simulink model "SO_SMC"  (R2023b)
settings: Solver=ode1  StartTime=0.0  StopTime=60  FixedStep=0.01  RelTol=1e-3
libraries: simulink x1
settings Model: Creator=vanch  LastModifiedBy=vanch

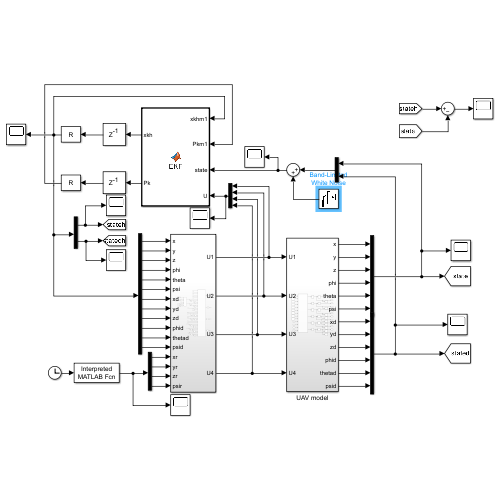
[thumbnail: Simulink's stored preview of the top-level diagram]
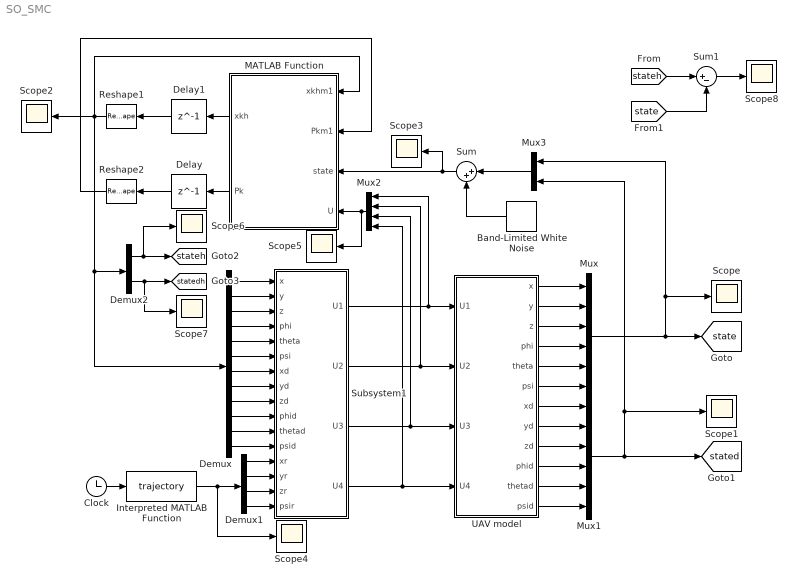
== system SO_SMC ==
  Band-Limited White Noise : simulink/Sources/Band-Limited White Noise  Cov=1e-8  Ts=0.01  seed=[1530]
  Clock : Clock
  Delay : Delay  DelayLength=1  InitialCondition=(1e-3)*eye(12,12)
  Delay1 : Delay  DelayLength=1  InitialCondition=0.001
  Demux : Demux  Outputs=12
  Demux1 : Demux
  Demux2 : Demux  Outputs=2
  Interpreted MATLAB Function : MATLABFcn  MATLABFcn=trajectory  OutputDimensions=4
  MATLAB Function : MATLAB Function  TreatAsAtomicUnit=on
  Mux : Mux  Inputs=6
  Mux1 : Mux  Inputs=6
  Mux2 : Mux
  Mux3 : Mux  Inputs=2
  Reshape1 : Reshape  OutputDimensionality=Customize  OutputDimensions=[12,1]
  Reshape2 : Reshape  OutputDimensionality=Customize  OutputDimensions=[12,12]
  Scope{,1..8} (9 alike) : Scope
  Subsystem1 : Subsystem
  Sum : Sum  Inputs=|++
  Sum1 : Sum  Inputs=|+-
  UAV model : Subsystem
  tag scope: state=global, stated=global, statedh=global, stateh=global
  wires:
  Mux/1 -> Mux3/1, Scope/1, [state]
  Subsystem1/1(U1) -> Mux2/1, UAV model/1(U1)
  UAV model/1(x) -> Mux/1
  UAV model/2(y) -> Mux/2
  UAV model/3(z) -> Mux/3
  UAV model/4(phi) -> Mux/4
  UAV model/5(theta) -> Mux/5
  UAV model/6(psi) -> Mux/6
  UAV model/7(xd) -> Mux1/1
  UAV model/8(yd) -> Mux1/2
  UAV model/9(zd) -> Mux1/3
  UAV model/10(phid) -> Mux1/4
  UAV model/11(thetad) -> Mux1/5
  UAV model/12(psid) -> Mux1/6
  Mux1/1 -> Mux3/2, Scope1/1, [stated]
  Mux2/1 -> Scope5/1, MATLAB Function/4(U)
  Sum/1 -> MATLAB Function/3(state), Scope3/1
  Mux3/1 -> Sum/1
  Delay1/1 -> Reshape1/1
  Delay/1 -> Reshape2/1
  Reshape2/1 -> MATLAB Function/2(Pkm1)
  MATLAB Function/1(xkh) -> Delay1/1
  MATLAB Function/2(Pk) -> Delay/1
  Demux/12 -> Subsystem1/12(psid)
  Demux/11 -> Subsystem1/11(thetad)
  Demux/10 -> Subsystem1/10(phid)
  Demux/9 -> Subsystem1/9(zd)
  Demux/8 -> Subsystem1/8(yd)
  Demux/7 -> Subsystem1/7(xd)
  Demux/6 -> Subsystem1/6(psi)
  Demux/5 -> Subsystem1/5(theta)
  Demux/4 -> Subsystem1/4(phi)
  Demux/3 -> Subsystem1/3(z)
  Demux/2 -> Subsystem1/2(y)
  Demux/1 -> Subsystem1/1(x)
  Subsystem1/2(U2) -> Mux2/2, UAV model/2(U2)
  Subsystem1/3(U3) -> Mux2/3, UAV model/3(U3)
  Subsystem1/4(U4) -> Mux2/4, UAV model/4(U4)
  Clock/1 -> Interpreted MATLAB Function/1
  Demux1/2 -> Subsystem1/14(yr)
  Demux1/4 -> Subsystem1/16(psir)
  Demux1/3 -> Subsystem1/15(zr)
  Demux1/1 -> Subsystem1/13(xr)
  Interpreted MATLAB Function/1 -> Scope4/1, Demux1/1
  Demux2/2 -> Scope7/1, [statedh]
  Reshape1/1 -> MATLAB Function/1(xkhm1), Scope2/1, Demux2/1, Demux/1
  Demux2/1 -> Scope6/1, [stateh]
  Band-Limited White Noise/1 -> Sum/2
  Sum1/1 -> Scope8/1
  [stateh] -> Sum1/1
  [state] -> Sum1/2

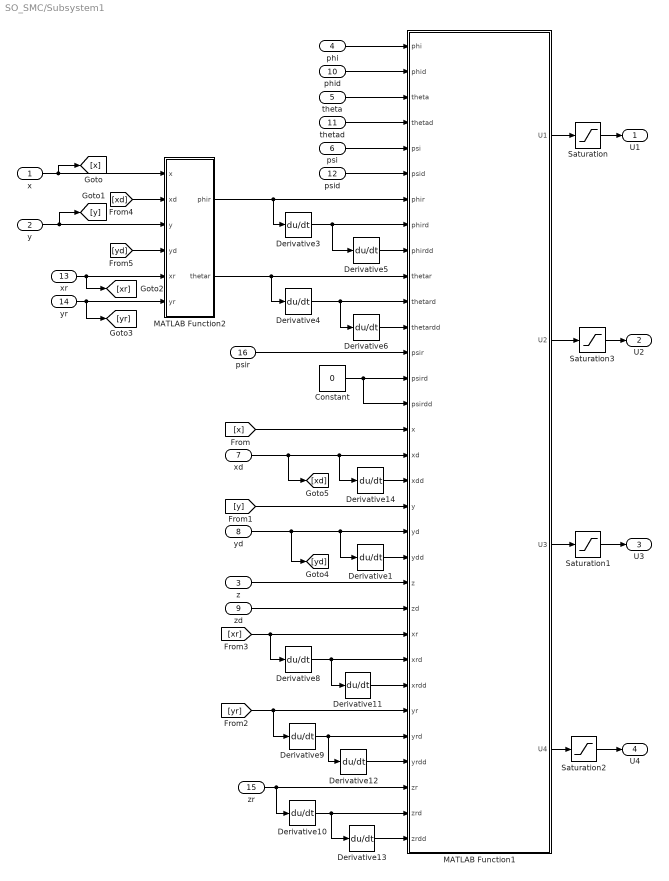
== system SO_SMC/Subsystem1 ==
  x : Inport
  y : Inport  Port=2
  z : Inport  Port=3
  phi : Inport  Port=4
  theta : Inport  Port=5
  psi : Inport  Port=6
  xd : Inport  Port=7
  yd : Inport  Port=8
  zd : Inport  Port=9
  phid : Inport  Port=10
  thetad : Inport  Port=11
  psid : Inport  Port=12
  xr : Inport  Port=13
  yr : Inport  Port=14
  zr : Inport  Port=15
  psir : Inport  Port=16
  Constant : Constant  Value=0
  Derivative{1,3..6,8..14} (12 alike) : Derivative
  MATLAB Function1 : MATLAB Function  TreatAsAtomicUnit=on
  MATLAB Function2 : MATLAB Function  TreatAsAtomicUnit=on
  Saturation : Saturate  UpperLimit=50  LowerLimit=0
  Saturation1 : Saturate  UpperLimit=0.01  LowerLimit=-0.01
  Saturation2 : Saturate  UpperLimit=0.01  LowerLimit=-0.01
  Saturation3 : Saturate  UpperLimit=0.01  LowerLimit=-0.01
  U1 : Outport
  U2 : Outport  Port=2
  U3 : Outport  Port=3
  U4 : Outport  Port=4
  wires:
  x/1 -> [x], MATLAB Function2/1(x)
  [yd] -> MATLAB Function2/4(yd)
  y/1 -> [y], MATLAB Function2/3(y)
  xr/1 -> [xr], MATLAB Function2/5(xr)
  yr/1 -> [yr], MATLAB Function2/6(yr)
  MATLAB Function2/1(phir) -> Derivative3/1, MATLAB Function1/7(phir)
  MATLAB Function2/2(thetar) -> MATLAB Function1/10(thetar), Derivative4/1
  Derivative3/1 -> MATLAB Function1/8(phird), Derivative5/1
  Derivative4/1 -> MATLAB Function1/11(thetard), Derivative6/1
  psir/1 -> MATLAB Function1/13(psir)
  [x] -> MATLAB Function1/16(x)
  [y] -> MATLAB Function1/19(y)
  xd/1 -> [xd], Derivative14/1, MATLAB Function1/17(xd)
  yd/1 -> [yd], MATLAB Function1/20(yd), Derivative1/1
  z/1 -> MATLAB Function1/22(z)
  zd/1 -> MATLAB Function1/23(zd)
  zr/1 -> MATLAB Function1/30(zr), Derivative10/1
  Derivative8/1 -> MATLAB Function1/25(xrd), Derivative11/1
  Derivative9/1 -> MATLAB Function1/28(yrd), Derivative12/1
  Derivative10/1 -> MATLAB Function1/31(zrd), Derivative13/1
  Derivative11/1 -> MATLAB Function1/26(xrdd)
  Derivative12/1 -> MATLAB Function1/29(yrdd)
  [yr] -> Derivative9/1, MATLAB Function1/27(yr)
  Derivative13/1 -> MATLAB Function1/32(zrdd)
  [xr] -> MATLAB Function1/24(xr), Derivative8/1
  MATLAB Function1/1(U1) -> Saturation/1
  [xd] -> MATLAB Function2/2(xd)
  Derivative6/1 -> MATLAB Function1/12(thetardd)
  Derivative5/1 -> MATLAB Function1/9(phirdd)
  psid/1 -> MATLAB Function1/6(psid)
  psi/1 -> MATLAB Function1/5(psi)
  thetad/1 -> MATLAB Function1/4(thetad)
  phid/1 -> MATLAB Function1/2(phid)
  Derivative1/1 -> MATLAB Function1/21(ydd)
  Derivative14/1 -> MATLAB Function1/18(xdd)
  Saturation/1 -> U1/1
  MATLAB Function1/4(U4) -> Saturation2/1
  theta/1 -> MATLAB Function1/3(theta)
  phi/1 -> MATLAB Function1/1(phi)
  MATLAB Function1/2(U2) -> Saturation3/1
  MATLAB Function1/3(U3) -> Saturation1/1
  Constant/1 -> MATLAB Function1/15(psirdd), MATLAB Function1/14(psird)
  Saturation3/1 -> U2/1
  Saturation1/1 -> U3/1
  Saturation2/1 -> U4/1

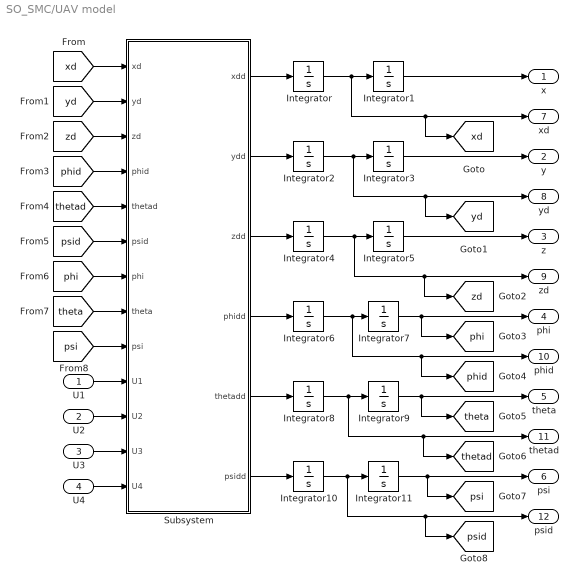
== system SO_SMC/UAV model ==
  U1 : Inport
  U2 : Inport  Port=2
  U3 : Inport  Port=3
  U4 : Inport  Port=4
  Integrator{,1..4,6..11} (11 alike) : Integrator  InitialCondition=0.01
  Integrator5 : Integrator  InitialCondition=0.01  LimitOutput=on  LowerSaturationLimit=0
  Subsystem : Subsystem
  x : Outport
  y : Outport  Port=2
  z : Outport  Port=3
  phi : Outport  Port=4
  theta : Outport  Port=5
  psi : Outport  Port=6
  xd : Outport  Port=7
  yd : Outport  Port=8
  zd : Outport  Port=9
  phid : Outport  Port=10
  thetad : Outport  Port=11
  psid : Outport  Port=12
  tag scope: phi=global, phid=global, psi=global, psid=global, theta=global, thetad=global, xd=global, yd=global, zd=global
  wires:
  Integrator5/1 -> z/1
  Integrator6/1 -> phid/1, [phid], Integrator7/1
  Integrator1/1 -> x/1
  [psid] -> Subsystem/6(psid)
  Integrator2/1 -> yd/1, [yd], Integrator3/1
  Subsystem/3(zdd) -> Integrator4/1
  Subsystem/6(psidd) -> Integrator10/1
  Integrator3/1 -> y/1
  Integrator8/1 -> thetad/1, [thetad], Integrator9/1
  [theta] -> Subsystem/8(theta)
  Integrator/1 -> xd/1, [xd], Integrator1/1
  [thetad] -> Subsystem/5(thetad)
  [zd] -> Subsystem/3(zd)
  Subsystem/4(phidd) -> Integrator6/1
  Integrator9/1 -> theta/1, [theta]
  [phid] -> Subsystem/4(phid)
  Integrator10/1 -> psid/1, [psid], Integrator11/1
  Subsystem/2(ydd) -> Integrator2/1
  Integrator4/1 -> zd/1, [zd], Integrator5/1
  Subsystem/5(thetadd) -> Integrator8/1
  Subsystem/1(xdd) -> Integrator/1
  [yd] -> Subsystem/2(yd)
  [psi] -> Subsystem/9(psi)
  Integrator11/1 -> psi/1, [psi]
  [xd] -> Subsystem/1(xd)
  [phi] -> Subsystem/7(phi)
  Integrator7/1 -> phi/1, [phi]
  U1/1 -> Subsystem/10(U1)
  U2/1 -> Subsystem/11(U2)
  U3/1 -> Subsystem/12(U3)
  U4/1 -> Subsystem/13(U4)

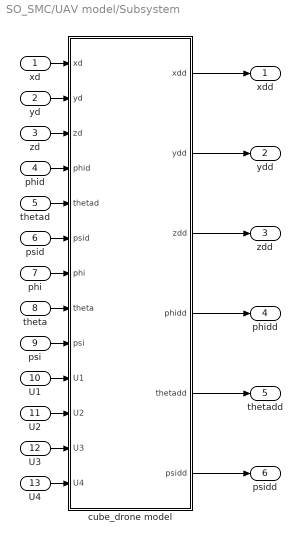
== system SO_SMC/UAV model/Subsystem ==
  xd : Inport
  yd : Inport  Port=2
  zd : Inport  Port=3
  phid : Inport  Port=4
  thetad : Inport  Port=5
  psid : Inport  Port=6
  phi : Inport  Port=7
  theta : Inport  Port=8
  psi : Inport  Port=9
  U1 : Inport  Port=10
  U2 : Inport  Port=11
  U3 : Inport  Port=12
  U4 : Inport  Port=13
  cube_drone model : MATLAB Function  TreatAsAtomicUnit=on
  xdd : Outport
  ydd : Outport  Port=2
  zdd : Outport  Port=3
  phidd : Outport  Port=4
  thetadd : Outport  Port=5
  psidd : Outport  Port=6
  wires:
  U4/1 -> cube_drone model/13(U4)
  U1/1 -> cube_drone model/10(U1)
  U2/1 -> cube_drone model/11(U2)
  cube_drone model/2(ydd) -> ydd/1
  cube_drone model/4(phidd) -> phidd/1
  U3/1 -> cube_drone model/12(U3)
  cube_drone model/3(zdd) -> zdd/1
  cube_drone model/5(thetadd) -> thetadd/1
  psid/1 -> cube_drone model/6(psid)
  cube_drone model/6(psidd) -> psidd/1
  zd/1 -> cube_drone model/3(zd)
  yd/1 -> cube_drone model/2(yd)
  thetad/1 -> cube_drone model/5(thetad)
  phid/1 -> cube_drone model/4(phid)
  phi/1 -> cube_drone model/7(phi)
  cube_drone model/1(xdd) -> xdd/1
  xd/1 -> cube_drone model/1(xd)
  theta/1 -> cube_drone model/8(theta)
  psi/1 -> cube_drone model/9(psi)

== matlab function SO_SMC/Subsystem1/MATLAB Function2 ==
  data: x input; phir output; xd input; thetar output; y input; yd input; xr input; yr input
function [phir,thetar] = fcn(x,xd,y,yd,xr,yr)
kpx=0.1;
kdx=0.15;
kpy=0.1;
kdy=0.15;
thetar=kpx*(xr-x)-kdx*xd;
phir=-kpy*(yr-y)+kdy*yd;
end

== matlab function SO_SMC/UAV model/Subsystem/cube_drone model ==
  data: xd input; xdd output; yd input; zd input; phid input; thetad input; psid input; phi input; theta input; psi input; U1 input; U2 input; U3 input; U4 input; ydd output; zdd output; phidd output; thetadd output; psidd output
function [xdd,ydd,zdd,phidd,thetadd,psidd] = fcn(xd,yd,zd,phid,thetad,psid,phi,theta,psi,U1,U2,U3,U4)
%cos,sin
cphi=cos(phi);
sphi=sin(phi);
ctheta=cos(theta);
stheta=sin(theta);
cpsi=cos(psi);
spsi=sin(psi);
%parameters
m=1.96;
g=9.81;
Kdx=0.00055670;
Kdy=0.00055670;
Kdz=0.0006354;
Ixx=0.00149;
Iyy=0.00153;
Izz=0.00532;
%motion equation
xdd=1/m*((spsi*sphi+cpsi*stheta*cphi)*U1-Kdx*xd);
ydd=1/m*((spsi*stheta*cphi-cpsi*sphi)*U1-Kdy*yd);
zdd=1/m*(ctheta*cphi*U1-Kdz*zd-m*g);
phidd=1/Ixx*(psid*thetad*(Iyy-Izz)+U2);
thetadd=1/Iyy*(psid*phid*(Izz-Ixx)+U3);
psidd=1/Izz*(phid*thetad*(Ixx-Iyy)+U4);
end

== matlab function SO_SMC/MATLAB Function ==
  data: xkhm1 input; Pkm1 input; xkh output; state input; U input; Pk output
function [xkh,Pk] = EKF(xkhm1,Pkm1,state,U)
%parameters
dt=0.01;
Q=1e-5;
R=1e-6;
m=1.96;
g=9.81;
Kdx=0.00055670;
Kdy=0.00055670;
Kdz=0.0006354;
Ixx=0.00149;
Iyy=0.00153;
Izz=0.00532;
%states
x=xkhm1(1);
y=xkhm1(2);
z=xkhm1(3);
phi=xkhm1(4);
theta=xkhm1(5);
psi=xkhm1(6);
xd=xkhm1(7);
yd=xkhm1(8);
zd=xkhm1(9);
phid=xkhm1(10);
thetad=xkhm1(11);
psid=xkhm1(12);
%linearized
A=[0, 0, 0, 0, 0, 0, 1, 0, 0, 0, 0, 0;
   0, 0, 0, 0, 0, 0, 0, 1, 0, 0, 0, 0;
   0, 0, 0, 0, 0, 0, 0, 0, 1, 0, 0, 0;
   0, 0, 0, 0, 0, 0, 0, 0, 0, 1, 0, 0;
   0, 0, 0, 0, 0, 0, 0, 0, 0, 0, 1, 0;
   0, 0, 0, 0, 0, 0, 0, 0, 0, 0, 0, 1;
   0, 0, 0, 0, 0, 0, -Kdx/m, 0, 0, 0, 0, 0;
  0, 0, 0, 0, 0, 0, 0, -Kdy/m, 0, 0, 0, 0;
  0, 0, 0, 0, 0, 0, 0, 0, -Kdz/m, 0, 0, 0;
  0, 0, 0, 0, 0, 0, 0, 0, 0, 0, (psid*(Iyy - Izz))/Ixx, (thetad*(Iyy - Izz))/Ixx;
  0, 0, 0, 0, 0, 0, 0, 0, 0, -(psid*(Ixx - Izz))/Iyy, 0, -(phid*(Ixx - Izz))/Iyy;
  0, 0, 0, 0, 0, 0, 0, 0, 0, (thetad*(Ixx - Iyy))/Izz, (phid*(Ixx - Iyy))/Izz, 0];
B=[0, 0, 0, 0;
   0, 0, 0, 0;
   0, 0, 0, 0;
   0, 0, 0, 0;
   0, 0, 0, 0;
   0, 0, 0, 0;
   (sin(phi)*sin(psi) + cos(phi)*cos(psi)*sin(theta))/m, 0, 0, 0;
   -(cos(psi)*sin(phi) - cos(phi)*sin(psi)*sin(theta))/m, 0, 0, 0;
   (cos(phi)*cos(theta))/m, 0, 0 ,0;
   0, 1/Ixx, 0, 0;
   0, 0, 1/Iyy, 0;
   0, 0, 0, 1/Izz];
%Prediction
xkhm=xkhm1+A*xkhm1*dt+B*U*dt;
Pkm=A*Pkm1*A'+Q*eye(12);
%update
Kk=(Pkm*eye(12))/(eye(12)*Pkm*eye(12)+R*eye(12));
xkh=xkhm+Kk*(state-eye(12)*xkhm);
Pk=(eye(12)-Kk*eye*(12))*Pkm;
end

== matlab function SO_SMC/Subsystem1/MATLAB Function1 ==
  data: phi input; phid input; theta input; thetad input; psi input; psid input; phir input; phird input; phirdd input; thetar input; thetard input; thetardd input; psir input; psird input; psirdd input; x input; U1 output; xd input; xdd input; y input; yd input; ydd input; z input; zd input; xr input; xrd input; xrdd input; yr input; yrd input; yrdd input; zr input; zrd input; zrdd input; U2 output; U3 output; U4 output
 function [U1,U2,U3,U4] = fcn(phi,phid,theta,thetad,psi,psid,phir,phird,phirdd,thetar,thetard,thetardd,psir,psird,psirdd,x,xd,xdd,y,yd,ydd,z,zd,xr,xrd,xrdd,yr,yrd,yrdd,zr,zrd,zrdd)
%paramters
m=1.96;
g=9.81;

Ixx=0.00149;
Iyy=0.00153;
Izz=0.00532;
Kdz=0.0006354;


epsilon1=1.7;
epsilon2=1.2;
epsilon3=1.5;
epsilon4=1.5;
eta1=2;
eta2=2;
eta3=5;
eta4=5;
cz=2.5;
cpsi=0.25;
c1=0.05;
c2=0.01;
c3=0.2;
c4=0.3;
c5=0.02;
c6=0.01;
c7=0.2;
c8=0.3;

d1=-Kdz*zd/m;
d3=psid*phid*(Izz-Ixx)/Iyy;
d4=thetad*psid*(Iyy-Izz)/Ixx;
d2=phid*thetad*(Ixx-Iyy)/Izz;
%functions


s1=cz*(zr-z)+(zrd-zd);
s2=cpsi*(psir-psi)+(psird-psid);
s3=c1*(xrd-xd)+c2*(xr-x)+c3*(thetard-thetad)+c4*(thetar-theta);
s4=c5*(yrd-yd)+c6*(yr-y)+c7*(phird-phid)+c8*(phir-phi);


U1=m*(cz*(zrd-zd)+zrdd+g-d1+epsilon1*sign(s1)+eta1*s1)/(cos(phi)*cos(theta));
U4=Izz*(cpsi*(psird-psid)-d2+psirdd+epsilon2*sign(s2)+eta2*s2);
U3=Iyy*(c1/c3*(xrdd-xdd)+c2/c3*(xrd-xd)+thetardd+c4/c3*(thetard-thetad)-d3+1/c3*(epsilon3*sign(s3)+eta3*s3));
U2=Ixx*(c5/c7*(yrdd-ydd)+c6/c7*(yrd-yd)+phirdd+c8/c7*(phird-phid)-d4+1/c7*(epsilon4*sign(s4)+eta4*s4));

end
